simulink model "EE192_Block_Diagram"  (R2017b)
settings: Solver=VariableStepAuto  StartTime=0.0  StopTime=10.0  RelTol=1e-3
settings Model: Creator=jrkro  LastModifiedBy=jrkro

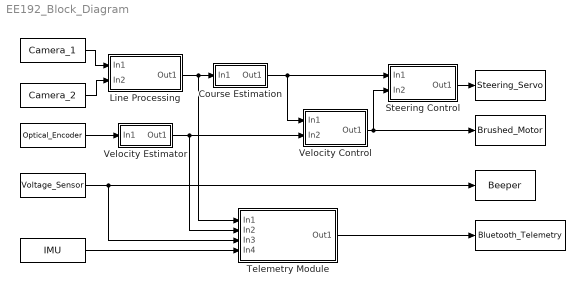
== system EE192_Block_Diagram ==
  " " : FromWorkspace  VariableName=Camera_1  SampleTime=0
  " " : FromWorkspace  VariableName=Optical_Encoder  SampleTime=0
  " " : FromWorkspace  VariableName=Camera_2  SampleTime=0
  " " : FromWorkspace  VariableName=IMU  SampleTime=0
  " " : FromWorkspace  VariableName=Voltage_Sensor  SampleTime=0
  " " : ToWorkspace  VariableName=Beeper  SaveFormat=Timeseries  SampleTime=-1
  " " : ToWorkspace  VariableName=Bluetooth_Telemetry  SaveFormat=Timeseries  SampleTime=-1
  " " : ToWorkspace  VariableName=Steering_Servo  SaveFormat=Timeseries  SampleTime=-1
  " " : ToWorkspace  VariableName=Brushed_Motor  SaveFormat=Timeseries  SampleTime=-1
  Course Estimation : Subsystem
  "Line Processing " : Subsystem
  Steering Control : Subsystem
  "Telemetry Module " : Subsystem
  Velocity Control : Subsystem
  Velocity Estimator : Subsystem
  wires:
  " "/1 -> "Line Processing "/1(In1)
  " "/1 -> "Line Processing "/2(In2)
  " "/1 -> "Telemetry Module "/3(In3), " "/1
  "Telemetry Module "/1(Out1) -> " "/1
  "Line Processing "/1(Out1) -> Course Estimation/1(In1), "Telemetry Module "/1(In1)
  Velocity Control/1(Out1) -> " "/1, Steering Control/2(In2)
  Steering Control/1(Out1) -> " "/1
  " "/1 -> Velocity Estimator/1(In1)
  Velocity Estimator/1(Out1) -> Velocity Control/2(In2), "Telemetry Module "/2(In2)
  " "/1 -> "Telemetry Module "/4(In4)
  Course Estimation/1(Out1) -> Steering Control/1(In1), Velocity Control/1(In1)

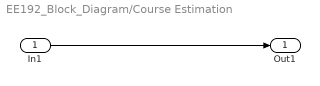
== system EE192_Block_Diagram/Course Estimation ==
  In1 : Inport
  Out1 : Outport
  wires:
  In1/1 -> Out1/1

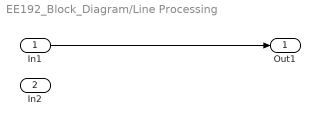
== system EE192_Block_Diagram/Line Processing  ==
  In1 : Inport
  In2 : Inport  Port=2
  Out1 : Outport
  wires:
  In1/1 -> Out1/1

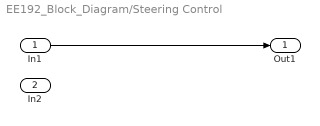
== system EE192_Block_Diagram/Steering Control ==
  In1 : Inport
  In2 : Inport  Port=2
  Out1 : Outport
  wires:
  In1/1 -> Out1/1

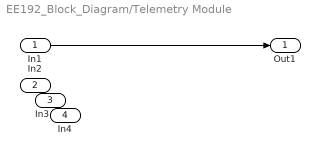
== system EE192_Block_Diagram/Telemetry Module  ==
  In1 : Inport
  In2 : Inport  Port=2
  In3 : Inport  Port=3
  In4 : Inport  Port=4
  Out1 : Outport
  wires:
  In1/1 -> Out1/1

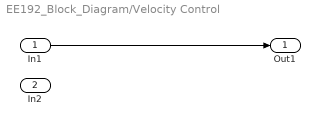
== system EE192_Block_Diagram/Velocity Control ==
  In1 : Inport
  In2 : Inport  Port=2
  Out1 : Outport
  wires:
  In1/1 -> Out1/1

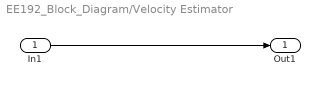
== system EE192_Block_Diagram/Velocity Estimator ==
  In1 : Inport
  Out1 : Outport
  wires:
  In1/1 -> Out1/1
